simulink model "InvertedPendulumSystem"  (R2023a)
settings: Solver=ode5  StartTime=0.0  StopTime=30  FixedStep=0.001  RelTol=1e-3
settings Model: Creator=zacha  LastModifiedBy=zacha

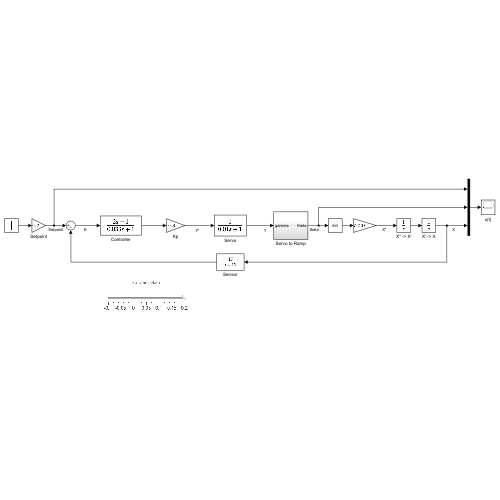
[thumbnail: Simulink's stored preview of the top-level diagram]
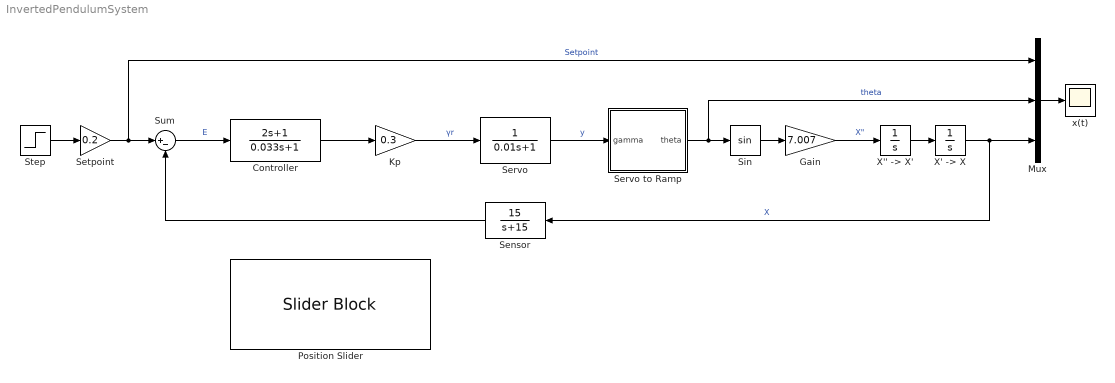
== system InvertedPendulumSystem ==
  Controller : TransferFcn  Numerator=[2 1]  Denominator=[0.033 1]
  Gain : Gain  Gain=7.007
  Kp : Gain  Gain=0.3
  Mux : Mux  Inputs=3
  Position Slider : SliderBlock  ScaleMin=-0.1  ScaleMax=0.2
  Sensor : TransferFcn  Numerator=[15]  Denominator=[1 15]
  Servo : TransferFcn  Denominator=[0.01 1]
  Servo to Ramp : Subsystem
  Setpoint : Gain  Gain=0.2
  Sin : Trigonometry
  Step : Step  Time=0  SampleTime=0
  Sum : Sum  Inputs=|+-
  "X' -> X" : Integrator
  "X'' -> X'" : Integrator
  x(t) : Scope
  wires:
  Step/1 -> Setpoint/1
  Sum/1 -> Controller/1  "E"
  Setpoint/1 -> Mux/1, Sum/1  "Setpoint"
  Sensor/1 -> Sum/2
  Sin/1 -> Gain/1
  "X'' -> X'"/1 -> "X' -> X"/1
  Gain/1 -> "X'' -> X'"/1  "X\""
  "X' -> X"/1 -> Mux/3, Sensor/1  "X"
  Mux/1 -> x(t)/1
  Kp/1 -> Servo/1  "γr"
  Servo/1 -> Servo to Ramp/1(gamma)  "y"
  Servo to Ramp/1(theta) -> Mux/2, Sin/1  "theta"
  Controller/1 -> Kp/1

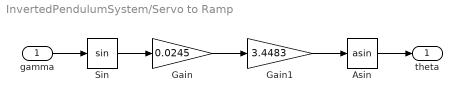
== system InvertedPendulumSystem/Servo to Ramp ==
  gamma : Inport
  Asin : Trigonometry  Operator=asin
  Gain : Gain  Gain=0.0245
  Gain1 : Gain  Gain=3.4483
  Sin : Trigonometry
  theta : Outport
  wires:
  Asin/1 -> theta/1
  Sin/1 -> Gain/1
  gamma/1 -> Sin/1
  Gain1/1 -> Asin/1
  Gain/1 -> Gain1/1
